simulink model "camera_capture_model"  (R2026a)
settings: Solver=VariableStepAuto  StopTime=5
values from neighbouring files (symbols this model uses):
  ego_pos = egoVehicle.Position    [loadSceneParams.m]
  target_pos = targetActor.Position    [loadSceneParams.m]
  target_speed = (target_pos_next - target_pos) / dt    [loadSceneParams.m]
undefined symbols (not defined in the file or in its folder): gray, Sim3dSensor
libraries: sim3dautolib x2, sim3dcameralib x1, sim3dlib x1
settings Model: Creator=The MathWorks, Inc.  LastModifiedBy=johnny
settings DebuggingCC: SymbolicDimsDataTypeCodeGenerationDiagnostic=none

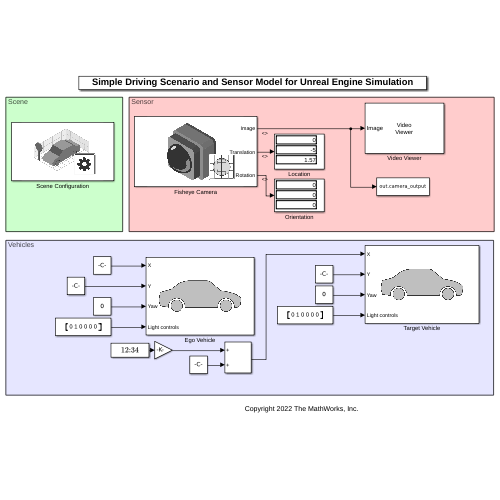
[thumbnail: Simulink's stored preview of the top-level diagram]
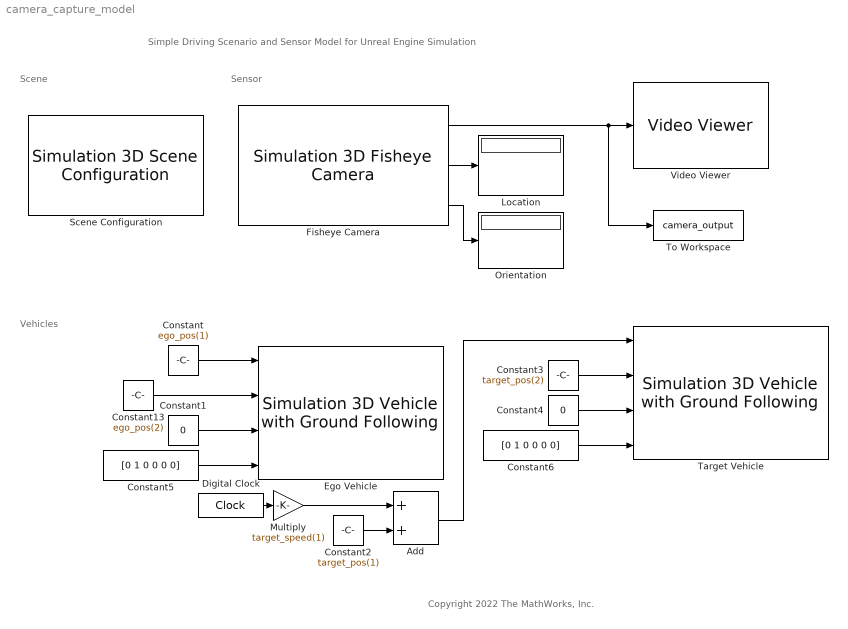
== system camera_capture_model ==
  note: Scene
  note: Copyright 2022 The MathWorks, Inc.
  note: Sensor
  note: Vehicles
  note: Simple Driving Scenario and Sensor Model for Unreal Engine Simulation
  Add : Sum
  Constant : Constant  Value=ego_pos(1)
  Constant1 : Constant  Value=0
  Constant13 : Constant  Value=ego_pos(2)
  Constant2 : Constant  Value=target_pos(1)
  Constant3 : Constant  Value=target_pos(2)
  Constant4 : Constant  Value=0
  Constant5 : Constant  Value=[0 1 0 0 0 0]
  Constant6 : Constant  Value=[0 1 0 0 0 0]
  Digital Clock : DigitalClock  SampleTime=0.01
  Ego Vehicle : sim3dautolib/Simulation 3D Vehicle with Ground Following  Priority=-1  PassVehMesh=Hatchback  MeshPath=/MathWorksSimulation/Vehicles/Muscle/Meshes/SK_MuscleCar.SK_MuscleCar  TrackWidth=1.9  WheelBase=3  WheelRadius=0.35  VehColor=Red  CoordinateSystem=ISO8855  InitialPos=[45, 0, 0]  InitialRot=[0, 0, 90]  ActorName=EgoVehicle  SampleTime=-1  ActorType=SimulinkVehicle  ID=C  aMode=3  ActorTag=EgoVehicle  CoordinateScheme=ISO  VehLightsControl=on  HeadlightColor=[ 1, 1, 1 ]  HighBeamIntensity=100000  LowBeamIntensity=60000  HighBeamConeAngle=70  LowBeamConeAngle=70  LeftHeadlightOrientation=[ 0, 0 ]  RightHeadlightOrientation=[ 0, 0 ]  BrakelightIntensity=500  ReverselightIntensity=500  SignallightIntensity=500  SignallightPeriod=1  SignalPulseWidth=50  TransformOutportEnabled=off
      settings: LibrarySourceBlock=drivingsim3d/Simulation 3D Vehicle with Ground Following
  Fisheye Camera : sim3dcameralib/Simulation 3D Fisheye Camera  Priority=1  sensorTag=Sim3dSensor�  sensorId=1  sensorName=Sim3dSensor�  vehTagList={'EgoVehicle';'Scene Origin';'TargetVehicle'}  vehTag=EgoVehicle  CoordinateSystem=ISO8855  mountLoc=Roof center  offsetFlag=off  tmountOffset=[0, 0, 0]  extTmount=off  rmountOffset=[0, 0, 0]  extRmount=off  OpticalCenter=[640, 360]  ImageSize=[720, 1280]  RadialDistortion=[320, -0.0005, 0, 0]  StretchMatrix=[1, 0; 0, 1]  TransformOutportEnabled=on  SampleTime=-1  mountPoint=[0 0 1.56]  mountOrientation=[0 0 0]  aMode=3  ID=1
      settings: LibrarySourceBlock=drivingsim3d/Simulation 3D Fisheye Camera
  Location : Display
  Multiply : Gain  Gain=target_speed(1)
  Orientation : Display
  Scene Configuration : sim3dlib/Simulation 3D Scene Configuration  Priority=0  ProjectFormat=Default Scenes  SceneDesc=Straight road  ProjectName=/usr/local/MATLAB/R2026a/toolbox/shared/sim3d_projects/automotive_project_linux/UE/LinuxNoEditor/VehicleSimulation.sh  ScenePath=/Game/Maps/HwStrght  EnableOpenDRIVE=off  vehTagList={'Custom';'EgoVehicle';'Scene Origin';'TargetVehicle'}  vehTag=EgoVehicle  AttachedCameraRelativeTranslation=[0 0 0]  FreeCameraDefaultInitialTranslation=[-6, 0, 2]  AttachedCameraRelativeRotation=[0, -15, 0]  FreeCameraDefaultInitialRotation=[0, -15, 0]  ViewpointName=Custom  FreeCameraInitialTranslation=[0 0 0]  FreeCameraInitialRotation=[0 0 0]  OpVisEn=off  Ts=0.1  EnableWindow=on  EnableRemoteAccess=off  SimulationMode=CoSimulation  SimulateUsing=Interpreted execution  EnableAnimationRecording=off  OverrideDefaultRecording=off  AnimationRecordingFileName=sim3dAnimation.mat  AnimationRecordingInterval=[0 inf]  EnableWeather=on  SunAzimuth=180.0  SunAltitude=0.0  EnableGeospatialSun=off  Latitude=0  Longitude=0  Date=2023-01-01  Time=10:30:00  GeoTimeZone=-5.0  SunDaylightSaving=off  wind=1  clouds=50.0  EnableVolumetricClouds=off  CloudCoverage=0  CloudAltitude=6  fog=0  rain=19.0  RaindropsEffect=off  SnowDensity=0  EnableGeospatial=off  TilesetSource=Earth terrain  UseTrueOrigin=off  OriginHeight=200  OriginLatitude=40.744652  OriginLongitude=-73.988864  MapStyle=Aerial  AdditionalAssetIDs=[]  UseAdvancedSunSky=off  SolarTime=11  TimeZone=-5  Day=21  Month=9  Year=2022  UseDaylightSavingTime=on  DSTStartDay=10  DSTStartMonth=3  DSTEndDay=3  DSTEndMonth=11  DSTSwitchHour=2  sensorTag=MainCamera2  sensorId=2  sensorName=MainCamera2  mountLoc=Origin  offsetFlag=off  tmountOffset=[0, 0, 0]  rmountOffset=[0, 0, 0]  HorizontalResolution=1280  VerticalResolution=720  HorizontalFOV=60  mountPoint=[0 0 0]  mountOrientation=[0 0 0]  aMode=3  ID=2  GeoTrigger=Inactive  ViewNameList={'Custom'}  ViewTranslationList={'[0 0 0]'}  ViewRotationList={'[0 0 0]'}
      settings: LibrarySourceBlock=drivingsim3d/Simulation 3D Scene Configuration
  Target Vehicle : sim3dautolib/Simulation 3D Vehicle with Ground Following  Priority=-1  PassVehMesh=Sport utility vehicle  MeshPath=/MathWorksSimulation/Vehicles/Muscle/Meshes/SK_MuscleCar.SK_MuscleCar  TrackWidth=1.9  WheelBase=3  WheelRadius=0.35  VehColor=Green  CoordinateSystem=ISO8855  InitialPos=[45, 10, 0]  InitialRot=[0, 0, 90]  ActorName=TargetVehicle  SampleTime=-1  ActorType=SimulinkVehicle  ID=C  aMode=3  ActorTag=TargetVehicle  CoordinateScheme=ISO  VehLightsControl=on  HeadlightColor=[ 1, 1, 1 ]  HighBeamIntensity=100000  LowBeamIntensity=60000  HighBeamConeAngle=70  LowBeamConeAngle=70  LeftHeadlightOrientation=[ 0, 0 ]  RightHeadlightOrientation=[ 0, 0 ]  BrakelightIntensity=500  ReverselightIntensity=500  SignallightIntensity=500  SignallightPeriod=1  SignalPulseWidth=50  TransformOutportEnabled=off
      settings: LibrarySourceBlock=drivingsim3d/Simulation 3D Vehicle with Ground Following
  To Workspace : ToWorkspace  VariableName=camera_output  SaveFormat=Structure With Time  SampleTime=-1
  Video Viewer : VideoViewer  colormapValue=gray(256)  FigPos=[893.8 568 530.4 430]
  wires:
  Multiply/1 -> Add/1
  Constant/1 -> Ego Vehicle/1
  Constant1/1 -> Ego Vehicle/3
  Constant2/1 -> Add/2
  Add/1 -> Target Vehicle/1
  Digital Clock/1 -> Multiply/1
  Fisheye Camera/2 -> Location/1
  Fisheye Camera/3 -> Orientation/1
  Constant4/1 -> Target Vehicle/3
  Constant5/1 -> Ego Vehicle/4
  Constant6/1 -> Target Vehicle/4
  Constant13/1 -> Ego Vehicle/2
  Constant3/1 -> Target Vehicle/2
  Fisheye Camera/1 -> To Workspace/1, Video Viewer/1
